simulink model "test"  (R2017b)
settings: Solver=FixedStepDiscrete  StartTime=0.0  StopTime=Inf  FixedStep=Ts  RelTol=1e-3
PreLoadFcn:
  | Ts = 0.01;
PostLoadFcn:
  | , if any(exist('dsrtsu_mdlpostloadfcn', 'file') == [2, 3, 6]), try dsrtsu_mdlpostloadfcn('Execute', bdroot); catch fprintf('Error in PostLoadFcn (dsrtsu_mdlpostloadfcn) for model "%s":\n %s\n', bdroot, lasterr); end, end,
libraries: rtican x19, simulink x9, rti1401lib_adc_type4 x3
(part 3 of 6)

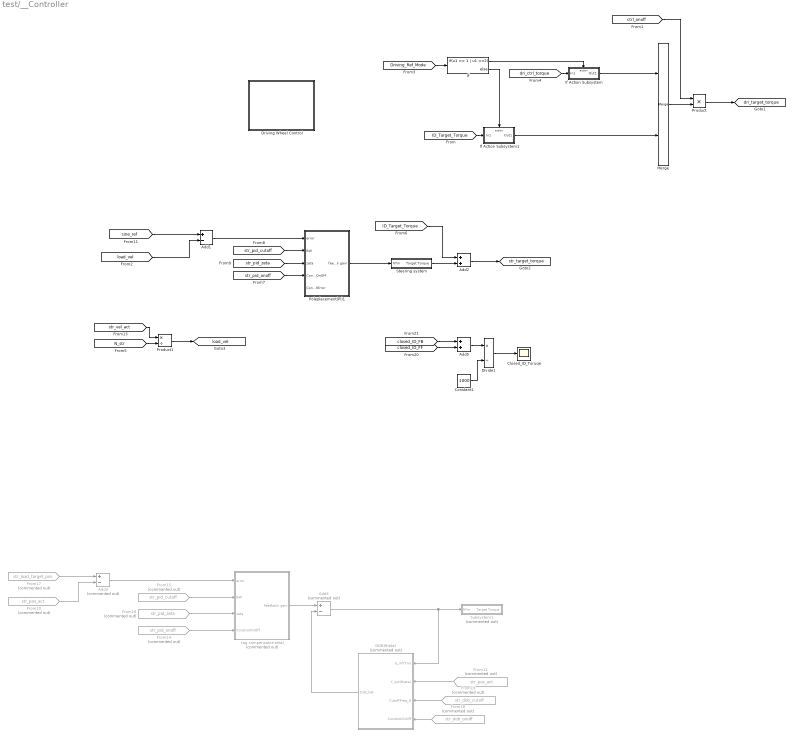
== system test/__Controller ==
  Add1 : Sum  Inputs=+-
  Add2 : Sum
  Add3 : Sum  Commented=on  Inputs=+-
  Add4 : Sum  Commented=on  Inputs=+-
  Add5 : Sum
  Closed_ID_Toruqe : Scope
  Constant1 : Constant  Value=1000
  DOB(theta) : Subsystem  Commented=on
  Divide1 : Product  Inputs=*/
  Driving Wheel Control : Subsystem
      mask Display: disp('Driving Wheel Control')
  From10 : From  Commented=on  GotoTag=str_pos_act  TagVisibility=global
  From12 : From  Commented=on  GotoTag=str_pos_act  TagVisibility=global
  From14 : From  Commented=on  GotoTag=str_pid_onoff  TagVisibility=global
  From15 : From  Commented=on  GotoTag=str_pid_cutoff  TagVisibility=global
  From16 : From  Commented=on  GotoTag=str_pid_zeta  TagVisibility=global
  From17 : From  Commented=on  GotoTag=str_load_target_pos  TagVisibility=global
  From18 : From  Commented=on  GotoTag=str_dob_onoff  TagVisibility=global
  From19 : From  Commented=on  GotoTag=str_dob_cutoff  TagVisibility=global
  If : If  IfExpression=u1 == 1 | u1 ==2
  If Action Subsystem : Subsystem  TreatAsAtomicUnit=on
  If Action Subsystem1 : Subsystem  TreatAsAtomicUnit=on
  Lag compensator(zeta) : Subsystem  Commented=on
  Merge : Merge
  Poleplacement(PI)1 : Subsystem
  Product : Product
  Product1 : Product  Inputs=*/
  Steering system : Subsystem
  Subsystem1 : Subsystem  Commented=on
  tag scope: dri_target_torque=global, load_vel=global, str_target_torque=global
  wires:
  If Action Subsystem1/1(Out1) -> Merge/2
  [dri_ctrl_torque] -> If Action Subsystem/1(In1)
  If/2 -> If Action Subsystem1/Action
  If/1 -> If Action Subsystem/Action
  [ID_Target_Torque] -> If Action Subsystem1/1(In1)
  [Driving_Ref_Mode] -> If/1
  If Action Subsystem/1(Out1) -> Merge/1
  [ctrl_onoff] -> Product/1
  Merge/1 -> Product/2
  Product/1 -> [dri_target_torque]
  [sine_ref] -> Add1/1
  [N_str] -> Product1/2
  [str_vel_act] -> Product1/1
  Add1/1 -> Poleplacement(PI)1/1(error)
  Poleplacement(PI)1/1(feedback gain) -> Steering system/1(N*m)
  Steering system/1(Target Torque) -> Add2/2
  Add2/1 -> [str_target_torque]
  [str_pid_onoff] -> Poleplacement(PI)1/4(ConstrolOnOff)
  [str_pid_cutoff] -> Poleplacement(PI)1/2(BW)
  [str_pid_zeta] -> Poleplacement(PI)1/3(zeta)
  Product1/1 -> [load_vel]
  [load_vel] -> Add1/2
  [ID_Target_Torque] -> Add2/1
  From10/1 -> Add3/2
  From17/1 -> Add3/1
  Add3/1 -> Lag compensator(zeta)/1(error)
  From15/1 -> Lag compensator(zeta)/2(BW)
  From16/1 -> Lag compensator(zeta)/3(zeta)
  From14/1 -> Lag compensator(zeta)/4(ConstrolOnOff)
  Lag compensator(zeta)/1(feedback gain) -> Add4/1
  DOB(theta)/1(Dist_hat) -> Add4/2
  Add4/1 -> Subsystem1/1(N*m), DOB(theta)/1(U_in*(Tm))
  From12/1 -> DOB(theta)/2(Y_out(theta))
  From18/1 -> DOB(theta)/4(ConstrolOnOff)
  From19/1 -> DOB(theta)/3(CutoffFreq_Q)
  [closed_ID_FF] -> Add5/2
  [closed_ID_FB] -> Add5/1
  Add5/1 -> Divide1/1
  Constant1/1 -> Divide1/2
  Divide1/1 -> Closed_ID_Toruqe/1

== system test/__Data Plotting ==
  ID_Target_Torque : Scope
  ID_idx : Scope
  __Drive_Ctrl_Plot : Subsystem
      mask Display: disp('Drive_Ctrl_Plot')
  __Motor_Feedback_Plot : Subsystem
      mask Display: disp('__Motor_Feedback_Plot')
  __Reference_Plot : Subsystem
      mask Display: disp('__Reference_Plot')
  __Sensor_Plot : Subsystem
      mask Display: disp('Sensor_Plot')
  wires:
  [ID_Target_Torque] -> ID_Target_Torque/1
  [ID_idx] -> ID_idx/1

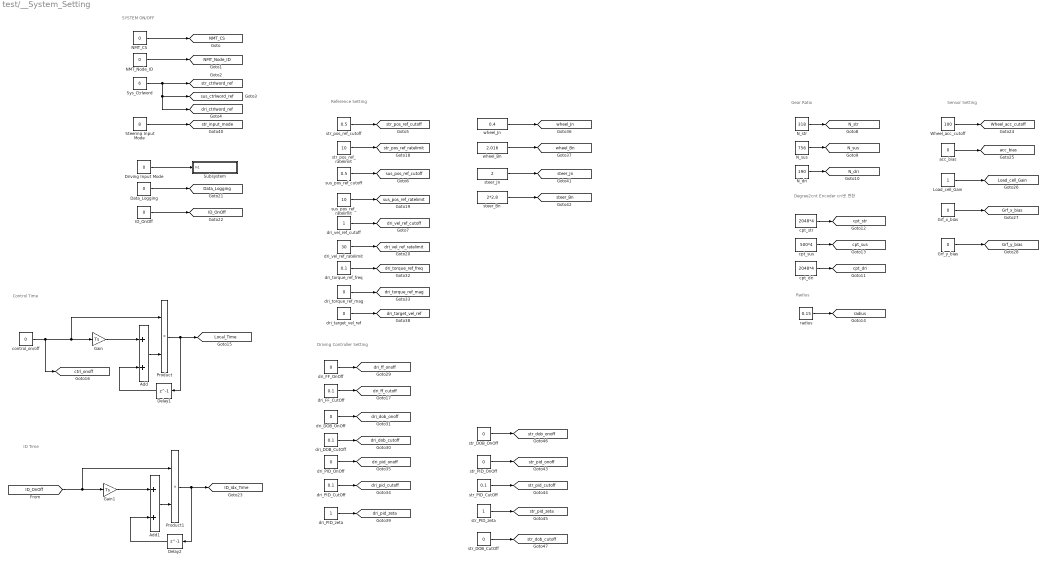
== system test/__System_Setting ==
  note: Driving Controller Setting
  note: Control Time
  note: Degree2cnt
      | Encoder cnt로 변환
  note: SYSTEM ON/OFF
  note: Gear Ratio
  note: Radius
  note: ID Time
  note: Reference Setting
  note: Sensor Setting
  Add : Sum
  Add1 : Sum
  Data_Logging : Constant  Value=0
  Delay1 : Delay  DelayLength=1  InitialCondition=0
  Delay2 : Delay  DelayLength=1  InitialCondition=0
  Driving Input Mode : Constant  Value=0
  Gain : Gain  Gain=Ts
  Gain1 : Gain  Gain=Ts
  Grf_x_bias : Constant  Value=0
  Grf_y_bias : Constant  Value=0
  ID_OnOff : Constant  Value=0
  Load_cell_Gain : Constant
  NMT_CS : Constant  Value=0
  NMT_Node_ID : Constant  Value=0
  N_dri : Constant  Value=190
  N_str : Constant  Value=318
  N_sus : Constant  Value=756
  Product : Product
  Product1 : Product
  Steering Input Mode : Constant  Value=8
  Subsystem : Subsystem
      mask Display: disp('Dri_Motor_Mode')
  Sys_Ctrlword : Constant  Value=6
  Wheel_acc_cutoff : Constant  Value=100
  acc_bias : Constant  Value=0
  control_on/off : Constant  Value=0
  cpt_dri : Constant  Value=2048*4
  cpt_str : Constant  Value=2048*4
  cpt_sus : Constant  Value=500*4
  dri_DOB_CutOff : Constant  Value=0.1
  dri_DOB_OnOff : Constant  Value=0
  dri_FF_CutOff : Constant  Value=0.1
  dri_FF_OnOff : Constant  Value=0
  dri_PID_CutOff : Constant  Value=0.1
  dri_PID_OnOff : Constant  Value=0
  dri_PID_zeta : Constant
  dri_target_vel_ref : Constant  Value=0
  dri_torque_ref_freq : Constant  Value=0.1
  dri_torque_ref_mag : Constant  Value=0
  dri_vel_ref_cutoff : Constant
  dri_vel_ref_ratelimit : Constant  Value=30
  radius : Constant  Value=0.15
  steer_Bn : Constant  Value=2*2.8
  steer_Jn : Constant  Value=2
  str_DOB_CutOff : Constant  Value=0
  str_DOB_OnOff : Constant  Value=0
  str_PID_CutOff : Constant  Value=0.1
  str_PID_OnOff : Constant  Value=0
  str_PID_zeta : Constant
  str_pos_ref_cutoff : Constant  Value=0.5
  str_pos_ref_ratelimit : Constant  Value=10
  sus_pos_ref_cutoff : Constant  Value=0.5
  sus_pos_ref_ratelimit : Constant  Value=10
  wheel_Bn : Constant  Value=2.016
  wheel_Jn : Constant  Value=0.4
  tag scope: Data_Logging=global, Grf_x_bias=global, Grf_y_bias=global, ID_OnOff=global, ID_idx_Time=global, Load_cell_Gain=global, Local_Time=global, NMT_CS=global, NMT_Node_ID=global, N_dri=global, N_str=global, N_sus=global, Wheel_acc_cutoff=global, acc_bias=global, cpt_dri=global, cpt_str=global, cpt_sus=global, ctrl_onoff=global, dri_ctrlword_ref=global, dri_dob_cutoff=global, dri_dob_onoff=global, dri_ff_cutoff=global, dri_ff_onoff=global, dri_pid_cutoff=global, dri_pid_onoff=global, dri_pid_zeta=global, dri_target_vel_ref=global, dri_torque_ref_freq=global, dri_torque_ref_mag=global, dri_vel_ref_cutoff=global, dri_vel_ref_ratelimit=global, radius=global, steer_Bn=global, steer_Jn=global, str_ctrlword_ref=global, str_dob_cutoff=global, str_dob_onoff=global, str_input_mode=global, str_pid_cutoff=global, str_pid_onoff=global, str_pid_zeta=global, str_pos_ref_cutoff=global, str_pos_ref_ratelimit=global, sus_ctrlword_ref=global, sus_pos_ref_cutoff=global, sus_pos_ref_ratelimit=global, wheel_Bn=global, wheel_Jn=global
  wires:
  NMT_CS/1 -> [NMT_CS]
  NMT_Node_ID/1 -> [NMT_Node_ID]
  Sys_Ctrlword/1 -> [dri_ctrlword_ref], [sus_ctrlword_ref], [str_ctrlword_ref]
  str_pos_ref_cutoff/1 -> [str_pos_ref_cutoff]
  sus_pos_ref_cutoff/1 -> [sus_pos_ref_cutoff]
  dri_vel_ref_cutoff/1 -> [dri_vel_ref_cutoff]
  N_str/1 -> [N_str]
  N_sus/1 -> [N_sus]
  N_dri/1 -> [N_dri]
  cpt_sus/1 -> [cpt_sus]
  cpt_dri/1 -> [cpt_dri]
  cpt_str/1 -> [cpt_str]
  radius/1 -> [radius]
  control_on/off/1 -> [ctrl_onoff], Product/1, Gain/1
  Gain/1 -> Add/1
  Add/1 -> Product/2
  Product/1 -> [Local_Time], Delay1/1
  Delay1/1 -> Add/2
  str_pos_ref_ratelimit/1 -> [str_pos_ref_ratelimit]
  sus_pos_ref_ratelimit/1 -> [sus_pos_ref_ratelimit]
  dri_vel_ref_ratelimit/1 -> [dri_vel_ref_ratelimit]
  Data_Logging/1 -> [Data_Logging]
  ID_OnOff/1 -> [ID_OnOff]
  Delay2/1 -> Add1/2
  Product1/1 -> [ID_idx_Time], Delay2/1
  [ID_OnOff] -> Product1/1, Gain1/1
  Gain1/1 -> Add1/1
  Add1/1 -> Product1/2
  Wheel_acc_cutoff/1 -> [Wheel_acc_cutoff]
  acc_bias/1 -> [acc_bias]
  Load_cell_Gain/1 -> [Load_cell_Gain]
  Grf_x_bias/1 -> [Grf_x_bias]
  Grf_y_bias/1 -> [Grf_y_bias]
  Driving Input Mode/1 -> Subsystem/1(In1)
  dri_DOB_OnOff/1 -> [dri_dob_onoff]
  dri_FF_CutOff/1 -> [dri_ff_cutoff]
  dri_DOB_CutOff/1 -> [dri_dob_cutoff]
  dri_FF_OnOff/1 -> [dri_ff_onoff]
  dri_torque_ref_mag/1 -> [dri_torque_ref_mag]
  dri_torque_ref_freq/1 -> [dri_torque_ref_freq]
  dri_PID_CutOff/1 -> [dri_pid_cutoff]
  dri_PID_OnOff/1 -> [dri_pid_onoff]
  wheel_Jn/1 -> [wheel_Jn]
  wheel_Bn/1 -> [wheel_Bn]
  dri_target_vel_ref/1 -> [dri_target_vel_ref]
  dri_PID_zeta/1 -> [dri_pid_zeta]
  Steering Input Mode/1 -> [str_input_mode]
  steer_Bn/1 -> [steer_Bn]
  steer_Jn/1 -> [steer_Jn]
  str_PID_OnOff/1 -> [str_pid_onoff]
  str_PID_CutOff/1 -> [str_pid_cutoff]
  str_PID_zeta/1 -> [str_pid_zeta]
  str_DOB_OnOff/1 -> [str_dob_onoff]
  str_DOB_CutOff/1 -> [str_dob_cutoff]

== system test/Hardware ActValue/Dot ==
  note: Dot
  in : Inport
  Sum1 : Sum  Inputs=+-  SaturateOnIntegerOverflow=on  InputSameDT=on  OutDataTypeStr=Inherit: Same as first input
  Sum2 : Sum  Inputs=+-  SaturateOnIntegerOverflow=on  InputSameDT=on  OutDataTypeStr=Inherit: Same as first input
  d : UnitDelay  SampleTime=Ts
  d1 : UnitDelay  SampleTime=Ts
  gain : Gain  Gain=2/Ts  SaturateOnIntegerOverflow=on  OutDataTypeStr=Inherit: Same as input  ParamDataTypeStr=Inherit: Same as input
  out : Outport
  wires:
  Sum1/1 -> d1/1, out/1
  d1/1 -> Sum1/2
  Sum2/1 -> gain/1
  in/1 -> d/1, Sum2/1
  d/1 -> Sum2/2
  gain/1 -> Sum1/1

== system test/Hardware ActValue/Driving Motor RX ==
  N30_TPDO0 : rtican/RTICAN Receive (RX)   Reserved1=[]  Reserved2=[]  Reserved3=[]  Reserved4=[]  SfcnMessage=[]  Msg_Struct=[]  BoardTypeNo=[]  BoardNo=[]  ChannelNo=[]  Parameters=[]  DialogFcn=[]  UnitName=[]  Revision=[]  UnitValues=[]  DSProperties=struct('RTI',struct('Version',uint32(5),'BlockType',struct('isSLSource',uint8(1),'isSLSink',uint8(1),'isHWSource',uint8(0),'isHWSink',uint8(0),'isSetup',uint8(0),'isInline',uint8(1),'isNonInline',uint8(0),'isInterrupt',uint8(0),'isChannelwise',uint8(0)),'IOBoardType','RTICAN','UnitType','MESSAGE','Identifier','RX','DialogType','MSVC','BlockSet','RTICAN','SlaveProcessor','CAN'))  RTIBlockInterface=struct('OutputPortsWidth',int32([1 1 1 1 1 1 1]),'OutputPortsActive',[1 1 1 1 1 1 1],'OutputPortsName',{{'Controlword','Statusword','Modes_of_operation_display','Error_code',['RX status'],['RX time'],['RX delta time']}},'OutputPortsDataType',{{'SS_DOUBLE','SS_DOUBLE','SS_DOUBLE','SS_DOUBLE','SS_DOUBLE','SS_DOUBLE','SS_DOUBLE'}},'OutputPortsLabel',{{'Controlword','Statusword','Modes_of_operation_display','Error_code','','',''}},'OutputPortsLabelMode','ON','InputPortsWidth',int32(0),'InputPortsActive',0,'DialogFcn','rtican_message_interface_gui','BlockDisplay',{{'','center'}},'IconTransparency','on','ParameterTunableNames',{{}},'InitLevel',3,'BlockName',struct('Token',{{'N30_TPDO0'}}),'SampleTime',{{-1}},'TriggerPort',{{'none'}},'EnablePort',{{'none'}})  RTIBlockParameters=struct('BoardTypeNo',{{1,'OFF',[]}},'BoardNo',{{1,'ON',[1 16]}},'ChannelNo',{{1,'ON',[1 2]}},'Parameters',{{struct('DataFileSupport',struct('DataFileSelectedMaster',1,'DataFileSelectedLocal',1,'DataFileName','c:\users\user\desktop\ycm\rcp\can1_canopen.dbc|','DataFileDate',['16-7-2025 15:06:12'],'SelectedFile',['..\..\ycm\rcp\ycm_canopen_v1 .dbc'],'InterfaceFcn','rtican_dbc_file_parser'),'Options',struct('StatusSelected',1,'TimeSelected',1,'DeltaTimeSelected',1,'BytePortSelected',0,'MessageLengthSelected',0,'TriggerPort',struct('Selected',0,'TriggerType',0),'UserCoding',struct('Selected',0,'InterfaceFile','UserDecodingFile','FcnName','UserDecodeFcn','InportSelected',0,'InportWidth',1,'OutportSelected',0,'OutportWidth',1),'EnablePortSelected',0,'SignalOnPortnameSelected',1,'UseRXService',0),'Message',struct('MsgOnBlocknameSelected',1,'MsgName','N30_TPDO0','MsgIdFormat',0,'MsgId',817,'MsgLength',7,'NumSignals',4,'SampleTime',-1,'Signal',struct('SgnName',{'Controlword','Statusword','Modes_of_operation_display','Error_code'},'SgnStartBit',{0,16,32,40},'SgnLength',{16,16,8,16},'ByteLayout',{0,0,0,0},'Factor',{1,1,1,1},'Offset',{0,0,0,0},'SgnComment',{'','','',''},'SgnUnit',{'','','',''},'Min',{0,0,0,0},'Max',{0,0,0,0},'SgnType',{0,0,0,0},'SLDataType',{'SS_DOUBLE','SS_DOUBLE','SS_DOUBLE','SS_DOUBLE'},'DataType',{0,0,1,0},'ModeValue',{-1,-1,-1,-1}),'MsgIdNumFormat',0,'MsgComment',{{''}}),'Version',1.2,'general',struct('isFromLib',0)),'OFF',[]}},'GroupId',{{struct('Group',{{'RTICAN'}},'No',1,'Behavior',{{'NAMECHANGE'}},'BlockType',{{'SINK'}},'NameChangeFlag',0),'OFF',[]}},'SFcnRTICANMessage',{{struct('MsgType','RX','SFcnPortType','Scalar','MsgName','N30_TPDO0','MsgIdFormat','STD','MsgId',817,'MsgLength',7,'NumSignals',4,'SampleTime',-1,'Signal',struct('SgnName',{'Controlword','Statusword','Modes_of_operation_display','Error_code'},'SgnStartBit',{0,16,32,40},'SgnLength',{16,16,8,16},'ByteLayout',{['little endian'],['little endian'],['little endian'],['little endian']},'Factor',{1,1,1,1},'Offset',{0,0,0,0},'SgnType',{'standard','standard','standard','standard'},'SLDataType',{'SS_DOUBLE','SS_DOUBLE','SS_DOUBLE','SS_DOUBLE'},'DataType',{['unsigned int'],['unsigned int'],['signed int'],['unsigned int']},'ModeValue',{-1,-1,-1,-1}),'StatusSelected','yes','TimeSelected','yes','DeltaTimeSelected','yes','BytePortSelected','no','MessageLengthSelected','no','TriggerPort',struct('Selected','no','TriggerType',0),'UserCoding',struct('Selected','no','InterfaceFile','UserDecodingFile','FcnName','UserDecodeFcn','InportSelected','no','InportWidth',1,'OutportSelected','no','OutportWidth',1),'EnablePortSelected','no','UseRXService','no','BoardType','DS1','BoardNo',1,'ControllerNo',1),'OFF',[]}},'TLCFileName',{{'rtican_rx_message','OFF',[]}})  RTISFcnParameters=struct('SFcnRTICANMessage','struct','TLCFileName','char')  RTIBlockParaDefault=struct('BoardTypeNo',4302,'BoardNo',1,'ChannelNo',1,'Parameters',struct('DataFileSupport',struct('DataFileSelectedMaster',0,'DataFileSelectedLocal',0,'DataFileName','','DataFileDate','','SelectedFile',['<no file selected>']),'Options',struct('StatusSelected',1,'TimeSelected',1,'DeltaTimeSelected',1,'BytePortSelected',0,'MessageLengthSelected',0,'TriggerPort',struct('Selected',0,'TriggerType','rising'),'UserCoding',struct('Selected',0,'InterfaceFile','UserDecodingFile','FcnName','UserDecodeFcn','InportSelected',0,'InportWidth',1,'OutportSelected',0,'OutportWidth',1),'EnablePortSelected',0,'SignalOnPortnameSelected',1,'UseRXService',0),'Message',struct('MsgOnBlocknameSelected',0,'MsgName',['RX Message'],'MsgIdFormat',0,'MsgId',100,'MsgLength',8,'NumSignals',1,'SampleTime',-1,'Signal',struct('SgnName',['RX signal'],'SgnStartBit',0,'SgnLength',8,'SgnType',0,'ModeValue',-1,'DataType',0,'SLDataType','SS_DOUBLE','ByteLayout',0,'Factor',1,'Offset',0,'Min',0,'Max',255,'SgnComment',{{}},'SgnUnit',''),'MsgIdNumFormat',0,'MsgComment',{{''}}),'Version',1.2,'general',struct('isFromLib',1)),'GroupId',struct('Group',{{'RTICAN'}},'No',1,'Behavior',{{'NAMECHANGE'}},'BlockType',{{'SINK'}},'NameChangeFlag',0),'SFcnRTICANMessage',struct('MsgType','RX','MsgName',['RX Message'],'MsgIdFormat','STD','MsgId',100,'MsgLength',8,'NumSignals',1,'SampleTime',-1,'Signal',struct('SgnName',['RX signal'],'SgnStartBit',0,'SgnLength',8,'SgnType','standard','ModeValue',-1,'DataType',['unsigned int'],'ByteLayout',['little endian'],'SLDataType','SS_DOUBLE','Factor',1,'Offset',0),'StatusSelected','yes','TimeSelected','yes','DeltaTimeSelected','yes','BytePortSelected','no','MessageLengthSelected','no','EnablePortSelected','no','UserCoding',struct('Selected','no','InterfaceFile','UserDecodingFile','FcnName','UserDecodeFcn','InportSelected','no','InportWidth',1,'OutportSelected','no','OutportWidth',1),'TriggerPort',struct('Selected','no','TriggerType','rising'),'UseRXService','no','BoardType','DS4302','BoardNo',1,'ControllerNo',1,'SFcnPortType','Scalar'),'TLCFileName','rtican_rx_message')
      settings: AttributesFormatString=Group Id: RTICAN1\n  SourceProductName=dSPACE RTI CAN Blockset
  N30_TPDO2 : rtican/RTICAN Receive (RX)   Reserved1=[]  Reserved2=[]  Reserved3=[]  Reserved4=[]  SfcnMessage=[]  Msg_Struct=[]  BoardTypeNo=[]  BoardNo=[]  ChannelNo=[]  Parameters=[]  DialogFcn=[]  UnitName=[]  Revision=[]  UnitValues=[]  DSProperties=struct('RTI',struct('Version',uint32(5),'BlockType',struct('isSLSource',uint8(1),'isSLSink',uint8(1),'isHWSource',uint8(0),'isHWSink',uint8(0),'isSetup',uint8(0),'isInline',uint8(1),'isNonInline',uint8(0),'isInterrupt',uint8(0),'isChannelwise',uint8(0)),'IOBoardType','RTICAN','UnitType','MESSAGE','Identifier','RX','DialogType','MSVC','BlockSet','RTICAN','SlaveProcessor','CAN'))  RTIBlockInterface=struct('OutputPortsWidth',int32([1 1 1 1 1]),'OutputPortsActive',[1 1 1 1 1],'OutputPortsName',{{'Velocity_demand_value','Velocity_actual_value_averaged',['RX status'],['RX time'],['RX delta time']}},'OutputPortsDataType',{{'SS_DOUBLE','SS_DOUBLE','SS_DOUBLE','SS_DOUBLE','SS_DOUBLE'}},'OutputPortsLabel',{{'Velocity_demand_value','Velocity_actual_value_averaged','','',''}},'OutputPortsLabelMode','ON','InputPortsWidth',int32(0),'InputPortsActive',0,'DialogFcn','rtican_message_interface_gui','BlockDisplay',{{'','center'}},'IconTransparency','on','ParameterTunableNames',{{}},'InitLevel',3,'BlockName',struct('Token',{{'N30_TPDO2'}}),'SampleTime',{{-1}},'TriggerPort',{{'none'}},'EnablePort',{{'none'}})  RTIBlockParameters=struct('BoardTypeNo',{{1,'OFF',[]}},'BoardNo',{{1,'ON',[1 16]}},'ChannelNo',{{1,'ON',[1 2]}},'Parameters',{{struct('DataFileSupport',struct('DataFileSelectedMaster',1,'DataFileSelectedLocal',1,'DataFileName','c:\users\user\desktop\ycm\rcp\can1_canopen.dbc|','DataFileDate',['16-7-2025 15:06:12'],'SelectedFile',['..\..\ycm\rcp\ycm_canopen_v1 .dbc'],'InterfaceFcn','rtican_dbc_file_parser'),'Options',struct('StatusSelected',1,'TimeSelected',1,'DeltaTimeSelected',1,'BytePortSelected',0,'MessageLengthSelected',0,'TriggerPort',struct('Selected',0,'TriggerType',0),'UserCoding',struct('Selected',0,'InterfaceFile','UserDecodingFile','FcnName','UserDecodeFcn','InportSelected',0,'InportWidth',1,'OutportSelected',0,'OutportWidth',1),'EnablePortSelected',0,'SignalOnPortnameSelected',1,'UseRXService',0),'Message',struct('MsgOnBlocknameSelected',1,'MsgName','N30_TPDO2','MsgIdFormat',0,'MsgId',819,'MsgLength',8,'NumSignals',2,'SampleTime',-1,'Signal',struct('SgnName',{'Velocity_demand_value','Velocity_actual_value_averaged'},'SgnStartBit',{0,32},'SgnLength',{32,32},'ByteLayout',{0,0},'Factor',{1,1},'Offset',{0,0},'SgnComment',{'',''},'SgnUnit',{'',''},'Min',{0,0},'Max',{0,0},'SgnType',{0,0},'SLDataType',{'SS_DOUBLE','SS_DOUBLE'},'DataType',{1,1},'ModeValue',{-1,-1}),'MsgIdNumFormat',0,'MsgComment',{{''}}),'Version',1.2,'general',struct('isFromLib',0)),'OFF',[]}},'GroupId',{{struct('Group',{{'RTICAN'}},'No',1,'Behavior',{{'NAMECHANGE'}},'BlockType',{{'SINK'}},'NameChangeFlag',0),'OFF',[]}},'SFcnRTICANMessage',{{struct('MsgType','RX','SFcnPortType','Scalar','MsgName','N30_TPDO2','MsgIdFormat','STD','MsgId',819,'MsgLength',8,'NumSignals',2,'SampleTime',-1,'Signal',struct('SgnName',{'Velocity_demand_value','Velocity_actual_value_averaged'},'SgnStartBit',{0,32},'SgnLength',{32,32},'ByteLayout',{['little endian'],['little endian']},'Factor',{1,1},'Offset',{0,0},'SgnType',{'standard','standard'},'SLDataType',{'SS_DOUBLE','SS_DOUBLE'},'DataType',{['signed int'],['signed int']},'ModeValue',{-1,-1}),'StatusSelected','yes','TimeSelected','yes','DeltaTimeSelected','yes','BytePortSelected','no','MessageLengthSelected','no','TriggerPort',struct('Selected','no','TriggerType',0),'UserCoding',struct('Selected','no','InterfaceFile','UserDecodingFile','FcnName','UserDecodeFcn','InportSelected','no','InportWidth',1,'OutportSelected','no','OutportWidth',1),'EnablePortSelected','no','UseRXService','no','BoardType','DS1','BoardNo',1,'ControllerNo',1),'OFF',[]}},'TLCFileName',{{'rtican_rx_message','OFF',[]}})  RTISFcnParameters=struct('SFcnRTICANMessage','struct','TLCFileName','char')  RTIBlockParaDefault=struct('BoardTypeNo',4302,'BoardNo',1,'ChannelNo',1,'Parameters',struct('DataFileSupport',struct('DataFileSelectedMaster',0,'DataFileSelectedLocal',0,'DataFileName','','DataFileDate','','SelectedFile',['<no file selected>']),'Options',struct('StatusSelected',1,'TimeSelected',1,'DeltaTimeSelected',1,'BytePortSelected',0,'MessageLengthSelected',0,'TriggerPort',struct('Selected',0,'TriggerType','rising'),'UserCoding',struct('Selected',0,'InterfaceFile','UserDecodingFile','FcnName','UserDecodeFcn','InportSelected',0,'InportWidth',1,'OutportSelected',0,'OutportWidth',1),'EnablePortSelected',0,'SignalOnPortnameSelected',1,'UseRXService',0),'Message',struct('MsgOnBlocknameSelected',0,'MsgName',['RX Message'],'MsgIdFormat',0,'MsgId',100,'MsgLength',8,'NumSignals',1,'SampleTime',-1,'Signal',struct('SgnName',['RX signal'],'SgnStartBit',0,'SgnLength',8,'SgnType',0,'ModeValue',-1,'DataType',0,'SLDataType','SS_DOUBLE','ByteLayout',0,'Factor',1,'Offset',0,'Min',0,'Max',255,'SgnComment',{{}},'SgnUnit',''),'MsgIdNumFormat',0,'MsgComment',{{''}}),'Version',1.2,'general',struct('isFromLib',1)),'GroupId',struct('Group',{{'RTICAN'}},'No',1,'Behavior',{{'NAMECHANGE'}},'BlockType',{{'SINK'}},'NameChangeFlag',0),'SFcnRTICANMessage',struct('MsgType','RX','MsgName',['RX Message'],'MsgIdFormat','STD','MsgId',100,'MsgLength',8,'NumSignals',1,'SampleTime',-1,'Signal',struct('SgnName',['RX signal'],'SgnStartBit',0,'SgnLength',8,'SgnType','standard','ModeValue',-1,'DataType',['unsigned int'],'ByteLayout',['little endian'],'SLDataType','SS_DOUBLE','Factor',1,'Offset',0),'StatusSelected','yes','TimeSelected','yes','DeltaTimeSelected','yes','BytePortSelected','no','MessageLengthSelected','no','EnablePortSelected','no','UserCoding',struct('Selected','no','InterfaceFile','UserDecodingFile','FcnName','UserDecodeFcn','InportSelected','no','InportWidth',1,'OutportSelected','no','OutportWidth',1),'TriggerPort',struct('Selected','no','TriggerType','rising'),'UseRXService','no','BoardType','DS4302','BoardNo',1,'ControllerNo',1,'SFcnPortType','Scalar'),'TLCFileName','rtican_rx_message')
      settings: AttributesFormatString=Group Id: RTICAN1\n  SourceProductName=dSPACE RTI CAN Blockset
  N30_TPDO3 : rtican/RTICAN Receive (RX)   Reserved1=[]  Reserved2=[]  Reserved3=[]  Reserved4=[]  SfcnMessage=[]  Msg_Struct=[]  BoardTypeNo=[]  BoardNo=[]  ChannelNo=[]  Parameters=[]  DialogFcn=[]  UnitName=[]  Revision=[]  UnitValues=[]  DSProperties=struct('RTI',struct('Version',uint32(5),'BlockType',struct('isSLSource',uint8(1),'isSLSink',uint8(1),'isHWSource',uint8(0),'isHWSink',uint8(0),'isSetup',uint8(0),'isInline',uint8(1),'isNonInline',uint8(0),'isInterrupt',uint8(0),'isChannelwise',uint8(0)),'IOBoardType','RTICAN','UnitType','MESSAGE','Identifier','RX','DialogType','MSVC','BlockSet','RTICAN','SlaveProcessor','CAN'))  RTIBlockInterface=struct('OutputPortsWidth',int32([1 1 1 1 1]),'OutputPortsActive',[1 1 1 1 1],'OutputPortsName',{{'Current_demand_value','Current_actual_value_averaged',['RX status'],['RX time'],['RX delta time']}},'OutputPortsDataType',{{'SS_DOUBLE','SS_DOUBLE','SS_DOUBLE','SS_DOUBLE','SS_DOUBLE'}},'OutputPortsLabel',{{'Current_demand_value','Current_actual_value_averaged','','',''}},'OutputPortsLabelMode','ON','InputPortsWidth',int32(0),'InputPortsActive',0,'DialogFcn','rtican_message_interface_gui','BlockDisplay',{{'','center'}},'IconTransparency','on','ParameterTunableNames',{{}},'InitLevel',3,'BlockName',struct('Token',{{'N30_TPDO3'}}),'SampleTime',{{-1}},'TriggerPort',{{'none'}},'EnablePort',{{'none'}})  RTIBlockParameters=struct('BoardTypeNo',{{1,'OFF',[]}},'BoardNo',{{1,'ON',[1 16]}},'ChannelNo',{{1,'ON',[1 2]}},'Parameters',{{struct('DataFileSupport',struct('DataFileSelectedMaster',1,'DataFileSelectedLocal',1,'DataFileName','c:\users\user\desktop\ycm\rcp\can1_canopen.dbc|','DataFileDate',['16-7-2025 15:06:12'],'SelectedFile',['..\..\ycm\rcp\ycm_canopen_v1 .dbc'],'InterfaceFcn','rtican_dbc_file_parser'),'Options',struct('StatusSelected',1,'TimeSelected',1,'DeltaTimeSelected',1,'BytePortSelected',0,'MessageLengthSelected',0,'TriggerPort',struct('Selected',0,'TriggerType',0),'UserCoding',struct('Selected',0,'InterfaceFile','UserDecodingFile','FcnName','UserDecodeFcn','InportSelected',0,'InportWidth',1,'OutportSelected',0,'OutportWidth',1),'EnablePortSelected',0,'SignalOnPortnameSelected',1,'UseRXService',0),'Message',struct('MsgOnBlocknameSelected',1,'MsgName','N30_TPDO3','MsgIdFormat',0,'MsgId',820,'MsgLength',8,'NumSignals',2,'SampleTime',-1,'Signal',struct('SgnName',{'Current_demand_value','Current_actual_value_averaged'},'SgnStartBit',{0,32},'SgnLength',{32,32},'ByteLayout',{0,0},'Factor',{1,1},'Offset',{0,0},'SgnComment',{'',''},'SgnUnit',{'',''},'Min',{0,0},'Max',{0,0},'SgnType',{0,0},'SLDataType',{'SS_DOUBLE','SS_DOUBLE'},'DataType',{1,1},'ModeValue',{-1,-1}),'MsgIdNumFormat',0,'MsgComment',{{''}}),'Version',1.2,'general',struct('isFromLib',0)),'OFF',[]}},'GroupId',{{struct('Group',{{'RTICAN'}},'No',1,'Behavior',{{'NAMECHANGE'}},'BlockType',{{'SINK'}},'NameChangeFlag',0),'OFF',[]}},'SFcnRTICANMessage',{{struct('MsgType','RX','SFcnPortType','Scalar','MsgName','N30_TPDO3','MsgIdFormat','STD','MsgId',820,'MsgLength',8,'NumSignals',2,'SampleTime',-1,'Signal',struct('SgnName',{'Current_demand_value','Current_actual_value_averaged'},'SgnStartBit',{0,32},'SgnLength',{32,32},'ByteLayout',{['little endian'],['little endian']},'Factor',{1,1},'Offset',{0,0},'SgnType',{'standard','standard'},'SLDataType',{'SS_DOUBLE','SS_DOUBLE'},'DataType',{['signed int'],['signed int']},'ModeValue',{-1,-1}),'StatusSelected','yes','TimeSelected','yes','DeltaTimeSelected','yes','BytePortSelected','no','MessageLengthSelected','no','TriggerPort',struct('Selected','no','TriggerType',0),'UserCoding',struct('Selected','no','InterfaceFile','UserDecodingFile','FcnName','UserDecodeFcn','InportSelected','no','InportWidth',1,'OutportSelected','no','OutportWidth',1),'EnablePortSelected','no','UseRXService','no','BoardType','DS1','BoardNo',1,'ControllerNo',1),'OFF',[]}},'TLCFileName',{{'rtican_rx_message','OFF',[]}})  RTISFcnParameters=struct('SFcnRTICANMessage','struct','TLCFileName','char')  RTIBlockParaDefault=struct('BoardTypeNo',4302,'BoardNo',1,'ChannelNo',1,'Parameters',struct('DataFileSupport',struct('DataFileSelectedMaster',0,'DataFileSelectedLocal',0,'DataFileName','','DataFileDate','','SelectedFile',['<no file selected>']),'Options',struct('StatusSelected',1,'TimeSelected',1,'DeltaTimeSelected',1,'BytePortSelected',0,'MessageLengthSelected',0,'TriggerPort',struct('Selected',0,'TriggerType','rising'),'UserCoding',struct('Selected',0,'InterfaceFile','UserDecodingFile','FcnName','UserDecodeFcn','InportSelected',0,'InportWidth',1,'OutportSelected',0,'OutportWidth',1),'EnablePortSelected',0,'SignalOnPortnameSelected',1,'UseRXService',0),'Message',struct('MsgOnBlocknameSelected',0,'MsgName',['RX Message'],'MsgIdFormat',0,'MsgId',100,'MsgLength',8,'NumSignals',1,'SampleTime',-1,'Signal',struct('SgnName',['RX signal'],'SgnStartBit',0,'SgnLength',8,'SgnType',0,'ModeValue',-1,'DataType',0,'SLDataType','SS_DOUBLE','ByteLayout',0,'Factor',1,'Offset',0,'Min',0,'Max',255,'SgnComment',{{}},'SgnUnit',''),'MsgIdNumFormat',0,'MsgComment',{{''}}),'Version',1.2,'general',struct('isFromLib',1)),'GroupId',struct('Group',{{'RTICAN'}},'No',1,'Behavior',{{'NAMECHANGE'}},'BlockType',{{'SINK'}},'NameChangeFlag',0),'SFcnRTICANMessage',struct('MsgType','RX','MsgName',['RX Message'],'MsgIdFormat','STD','MsgId',100,'MsgLength',8,'NumSignals',1,'SampleTime',-1,'Signal',struct('SgnName',['RX signal'],'SgnStartBit',0,'SgnLength',8,'SgnType','standard','ModeValue',-1,'DataType',['unsigned int'],'ByteLayout',['little endian'],'SLDataType','SS_DOUBLE','Factor',1,'Offset',0),'StatusSelected','yes','TimeSelected','yes','DeltaTimeSelected','yes','BytePortSelected','no','MessageLengthSelected','no','EnablePortSelected','no','UserCoding',struct('Selected','no','InterfaceFile','UserDecodingFile','FcnName','UserDecodeFcn','InportSelected','no','InportWidth',1,'OutportSelected','no','OutportWidth',1),'TriggerPort',struct('Selected','no','TriggerType','rising'),'UseRXService','no','BoardType','DS4302','BoardNo',1,'ControllerNo',1,'SFcnPortType','Scalar'),'TLCFileName','rtican_rx_message')
      settings: AttributesFormatString=Group Id: RTICAN1\n  SourceProductName=dSPACE RTI CAN Blockset
  Controlword : Outport
  Statusword : Outport  Port=2
  Modes_of_operation_display : Outport  Port=3
  Error_code : Outport  Port=4
  Velocity_demand_value : Outport  Port=5
  Velocity_actual_value_averaged : Outport  Port=6
  Current_demand_value : Outport  Port=7
  Current_actual_value_averaged : Outport  Port=8
  wires:
  N30_TPDO3/1 -> Current_demand_value/1  "Current_demand_value"
  N30_TPDO3/2 -> Current_actual_value_averaged/1  "Current_actual_value_averaged"
  N30_TPDO2/1 -> Velocity_demand_value/1  "Velocity_demand_value"
  N30_TPDO2/2 -> Velocity_actual_value_averaged/1  "Velocity_actual_value_averaged"
  N30_TPDO0/1 -> Controlword/1  "Controlword"
  N30_TPDO0/2 -> Statusword/1  "Statusword"
  N30_TPDO0/3 -> Modes_of_operation_display/1  "Modes_of_operation_display"
  N30_TPDO0/4 -> Error_code/1  "Error_code"

== system test/Hardware ActValue/LPF ==
  note: LPF : tau = 1/(2*pi*fc)
  note: y(n) = [Ts*{x(n)+x(n-1)}+(2*tau-Ts)*y(n-1)]/(2*tau+Ts)
  note: H(s) = 1/(tau*s+1)
  note: s = 2/Ts*(z-1)/(z+1)
  In : Inport
  fc : Inport  Port=2
  Constant : Constant  Value=Ts  SampleTime=Ts
  Constant1 : Constant  SampleTime=Ts
  Product1 : Product  Inputs=*/  RndMeth=Zero
  Product11 : Product  RndMeth=Zero
  Product2 : Product  Inputs=*/  RndMeth=Zero
  Sum1 : Sum  Inputs=+-  SaturateOnIntegerOverflow=on  InputSameDT=on  OutDataTypeStr=Inherit: Same as first input
  Sum2 : Sum  SaturateOnIntegerOverflow=on  InputSameDT=on  OutDataTypeStr=Inherit: Same as first input
  Sum3 : Sum  SaturateOnIntegerOverflow=on  InputSameDT=on  OutDataTypeStr=Inherit: Same as first input
  Sum4 : Sum  SaturateOnIntegerOverflow=on  InputSameDT=on  OutDataTypeStr=Inherit: Same as first input
  d : UnitDelay  SampleTime=Ts
  d1 : UnitDelay  SampleTime=Ts
  gain : Gain  Gain=Ts  SaturateOnIntegerOverflow=on  OutDataTypeStr=Inherit: Same as input  ParamDataTypeStr=Inherit: Same as input
  gain1 : Gain  Gain=2  SaturateOnIntegerOverflow=on  OutDataTypeStr=Inherit: Same as input  ParamDataTypeStr=Inherit: Same as input
  gain2 : Gain  Gain=2*pi  SaturateOnIntegerOverflow=on  OutDataTypeStr=Inherit: Same as input  ParamDataTypeStr=Inherit: Same as input
  Out : Outport
  wires:
  In/1 -> Sum3/1, d1/1
  d1/1 -> Sum3/2
  Sum3/1 -> gain/1
  gain/1 -> Sum2/1
  Product11/1 -> Sum2/2
  Sum1/1 -> Product11/1
  Constant/1 -> Sum1/2, Sum4/2
  fc/1 -> gain2/1
  gain1/1 -> Sum1/1, Sum4/1
  d/1 -> Product11/2
  Sum2/1 -> Product1/1
  Sum4/1 -> Product1/2
  Product1/1 -> Out/1, d/1
  Product2/1 -> gain1/1
  Constant1/1 -> Product2/1
  gain2/1 -> Product2/2
